simulink model "LightControlSWC"  (R2022b)
settings: Solver=FixedStepDiscrete  StartTime=0.0  StopTime=10.0  FixedStep=0.001  RelTol=1e-3
undefined symbols (not defined in the file): DESetLightState, OPSetLightState
settings Model: Creator=Lenovo  LastModifiedBy=Lenovo
settings OptimizationCC: DefaultParameterBehavior=Inlined  EnhancedBackFolding=on  PassReuseOutputArgsAs=Individual arguments  ZeroExternalMemoryAtStartup=off  ZeroInternalMemoryAtStartup=off  OptimizeBlockOrder=speed  DifferentSizesBufferReuse=on  OptimizationCustomize=off  EfficientTunableParamExpr=on
settings DebuggingCC: ParameterTunabilityLossMsg=error
settings SFSimCC: MATLABDynamicMemAlloc=off
settings RTWCC: Description=AUTOSAR  SystemTargetFile=autosar.tlc  GenCodeOnly=on  TemplateMakefile=ert_default_tmf
settings CodeAppCC: ForceParamTrailComments=on  IgnoreCustomStorageClasses=off  OperatorAnnotations=on  SimulinkDataObjDesc=on  SFDataObjDesc=on  InsertBlockDesc=on
settings STFCustomTargetCC: TargetLangStandard=C99 (ISO)  MultiwordLength=256  ParMdlRefBuildCompliant=on  CompOptLevelCompliant=on  IncludeMdlTerminateFcn=off  CombineOutputUpdateFcns=on  SuppressErrorStatus=on  ERTCustomFileBanners=on  SupportNonFinite=off  SupportComplex=off  SupportContinuousTime=off  SupportNonInlinedSFcns=off  RemoveResetFunc=on  MATLABClassNameForMDSCustomization=Simulink.SoftwareTarget.ERTCustomization  AutosarCompliant=on  UseToolchainInfoCompliant=on  LookupTableObjectStructAxisOrder=2,1,3,4,...  LUTObjectStructOrderEvenSpacing=Size,Table,Breakpoints  SystemTargetFile=autosar.tlc
settings ERTTargetCC: TargetLangStandard=C99 (ISO)  ConcurrentExecutionCompliant=off  IncludeMdlTerminateFcn=off  SuppressErrorStatus=on  SupportNonFinite=off  SupportComplex=off  ModelStepFunctionPrototypeControlCompliant=off  CPPClassGenCompliant=off  AutosarCompliant=on  LookupTableObjectStructAxisOrder=2,1,3,4,...  LUTObjectStructOrderEvenSpacing=Size,Table,Breakpoints  InlinedParameterPlacement=NonHierarchical  ERTCustomFileTemplate=example_file_process.tlc

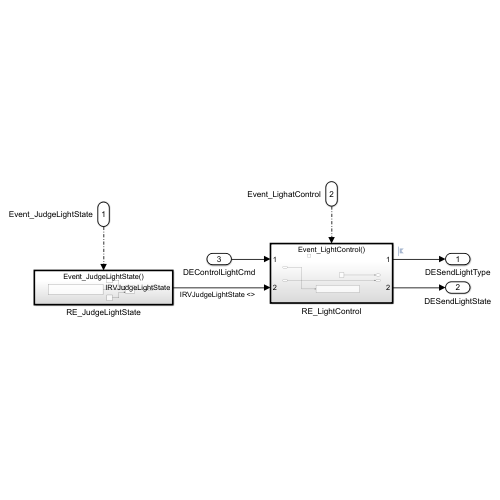
[thumbnail: Simulink's stored preview of the top-level diagram]
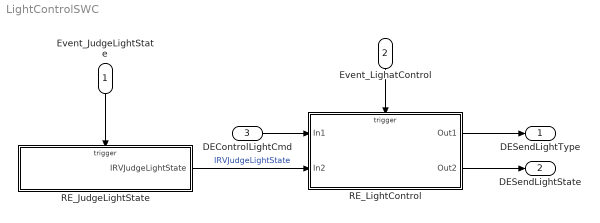
== system LightControlSWC ==
  Event_JudgeLightState : Inport  SampleTime=0.02  OutputFunctionCall=on
  Event_LighatControl : Inport  Port=2  OutputFunctionCall=on
  DEControlLightCmd : Inport  Port=3
  RE_JudgeLightState : Subsystem  TreatAsAtomicUnit=on
  RE_LightControl : Subsystem  TreatAsAtomicUnit=on
  DESendLightType : Outport
  DESendLightState : Outport  Port=2
  wires:
  RE_LightControl/1(Out1) -> DESendLightType/1
  RE_LightControl/2(Out2) -> DESendLightState/1
  DEControlLightCmd/1 -> RE_LightControl/1(In1)
  RE_JudgeLightState/1(IRVJudgeLightState) -> RE_LightControl/2(In2)  "IRVJudgeLightState"
  Event_LighatControl/1 -> RE_LightControl/Trigger
  Event_JudgeLightState/1 -> RE_JudgeLightState/Trigger

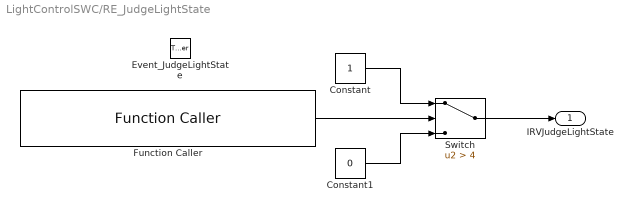
== system LightControlSWC/RE_JudgeLightState ==
  Event_JudgeLightState : TriggerPort  TriggerType=function-call  VariantControl=(inherit)
  Constant : Constant
  Constant1 : Constant  Value=0
  Function Caller : FunctionCaller  FunctionPrototype=DEGetLightState = OPGetLightState()  InputArgumentSpecifications=<Enter example>  OutputArgumentSpecifications=uint8(1)
  Switch : Switch  Criteria=u2 > Threshold  Threshold=4  OutDataTypeStr=int8  SaturateOnIntegerOverflow=off  InputSameDT=off
  IRVJudgeLightState : Outport  OutDataTypeStr=int8
  wires:
  Function Caller/1 -> Switch/2
  Constant1/1 -> Switch/3
  Constant/1 -> Switch/1
  Switch/1 -> IRVJudgeLightState/1

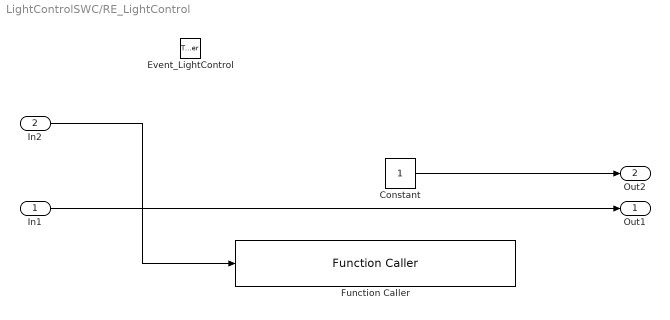
== system LightControlSWC/RE_LightControl ==
  In1 : Inport
  In2 : Inport  Port=2
  Event_LightControl : TriggerPort  TriggerType=function-call  VariantControl=(inherit)
  Constant : Constant
  Function Caller : FunctionCaller  FunctionPrototype=OPSetLightState(DESetLightState)  InputArgumentSpecifications=int8(1)  OutputArgumentSpecifications=<Enter example>
  Out1 : Outport
  Out2 : Outport  Port=2
  wires:
  In1/1 -> Out1/1
  In2/1 -> Function Caller/1
  Constant/1 -> Out2/1
